simulink model "internal_system"  (R2022b)
settings: Solver=VariableStepAuto  StartTime=0.0  StopTime=600  RelTol=1e-3
model workspace (MAT data in the model file):
  F = 1
settings Model: Creator=aless  LastModifiedBy=aless
settings DebuggingCC: UnconnectedInputMsg=warning  UnconnectedOutputMsg=warning  UnconnectedLineMsg=warning
settings ModelReferenceCC: EnableRefExpFcnMdlSchedulingChecks=on
settings RTWCC: DLArmComputeVersion=19.05

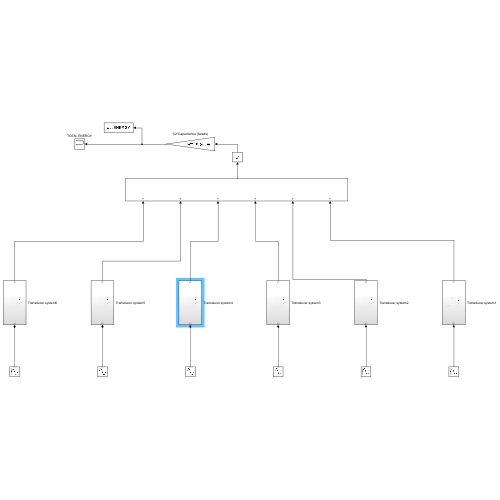
[thumbnail: Simulink's stored preview of the top-level diagram]
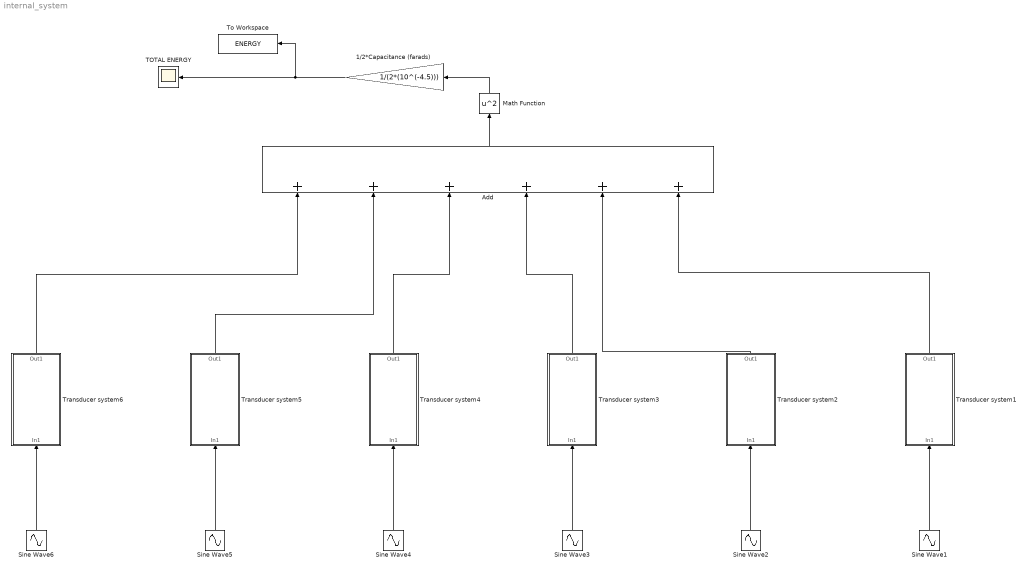
== system internal_system ==
  1/2*Capacitance (farads) : Gain  Gain=1/(2*(10^(-4.5)))
  Add : Sum  Inputs=++++++
  Math Function : Math  Operator=square
  Sine Wave1 : Sin  Amplitude=18670  Frequency=0.1176  SampleTime=0
  Sine Wave2 : Sin  Amplitude=18670  Frequency=0.1176  Phase=1/2  SampleTime=0
  Sine Wave3 : Sin  Amplitude=18670  Frequency=0.1176  Phase=1/3  SampleTime=0
  Sine Wave4 : Sin  Amplitude=18670  Frequency=0.1176  Phase=4/5  SampleTime=0
  Sine Wave5 : Sin  Amplitude=18670  Frequency=0.1176  Phase=1/5  SampleTime=0
  Sine Wave6 : Sin  Amplitude=18670  Frequency=0.1176  Phase=11/12  SampleTime=0
  TOTAL ENERGY : Scope
  To Workspace : ToWorkspace  VariableName=ENERGY  SaveFormat=Timeseries  SampleTime=-1
  Transducer system1 : Subsystem
  Transducer system2 : Subsystem
  Transducer system3 : Subsystem
  Transducer system4 : Subsystem
  Transducer system5 : Subsystem
  Transducer system6 : Subsystem
  wires:
  Sine Wave5/1 -> Transducer system5/1(In1)
  Sine Wave4/1 -> Transducer system4/1(In1)
  Sine Wave3/1 -> Transducer system3/1(In1)
  Sine Wave2/1 -> Transducer system2/1(In1)
  Sine Wave1/1 -> Transducer system1/1(In1)
  Transducer system6/1(Out1) -> Add/1
  Transducer system5/1(Out1) -> Add/2
  Transducer system4/1(Out1) -> Add/3
  Sine Wave6/1 -> Transducer system6/1(In1)
  Transducer system1/1(Out1) -> Add/6
  Transducer system2/1(Out1) -> Add/5
  Transducer system3/1(Out1) -> Add/4
  1/2*Capacitance (farads)/1 -> To Workspace/1, TOTAL ENERGY/1
  Add/1 -> Math Function/1
  Math Function/1 -> 1/2*Capacitance (farads)/1

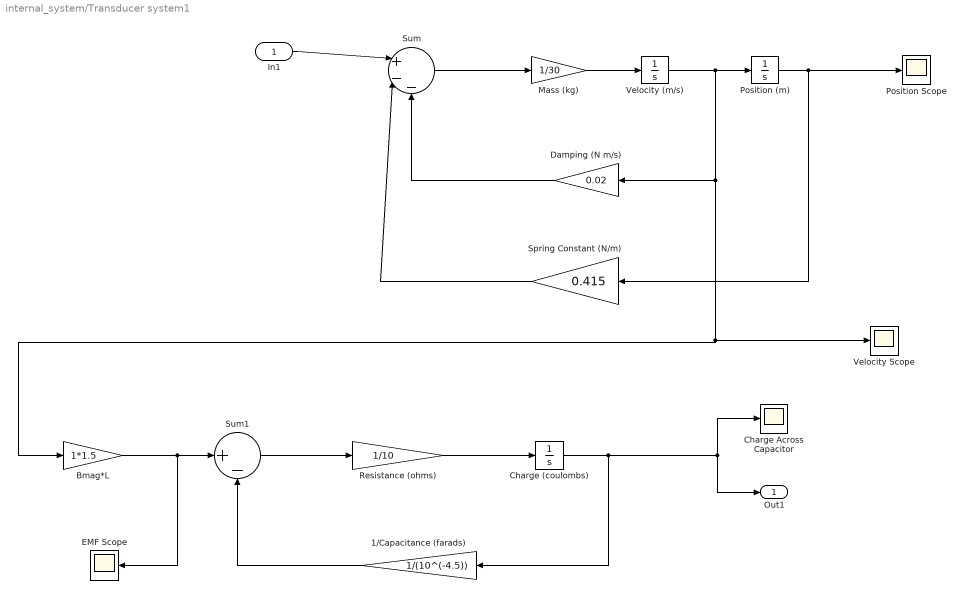
== system internal_system/Transducer system1 ==
  In1 : Inport
  1/Capacitance (farads) : Gain  Gain=1/(10^(-4.5))
  Bmag*L : Gain  Gain=1*1.5
  Charge (coulombs) : Integrator
  Charge Across Capacitor : Scope
  Damping (N m/s) : Gain  Gain=0.02
  EMF Scope : Scope
  Mass (kg) : Gain  Gain=1/30
  Position (m) : Integrator
  Position Scope : Scope
  Resistance (ohms) : Gain  Gain=1/10
  Spring Constant (N/m) : Gain  Gain=0.415
  Sum : Sum  Inputs=|+--
  Sum1 : Sum  Inputs=|+-
  Velocity (m/s) : Integrator
  Velocity Scope : Scope
  Out1 : Outport
  wires:
  Mass (kg)/1 -> Velocity (m/s)/1
  Sum/1 -> Mass (kg)/1
  Damping (N m/s)/1 -> Sum/3
  Position (m)/1 -> Position Scope/1, Spring Constant (N/m)/1
  Spring Constant (N/m)/1 -> Sum/2
  Velocity (m/s)/1 -> Damping (N m/s)/1, Bmag*L/1, Velocity Scope/1, Position (m)/1
  In1/1 -> Sum/1
  Sum1/1 -> Resistance (ohms)/1
  Bmag*L/1 -> EMF Scope/1, Sum1/1
  1/Capacitance (farads)/1 -> Sum1/2
  Resistance (ohms)/1 -> Charge (coulombs)/1
  Charge (coulombs)/1 -> 1/Capacitance (farads)/1, Out1/1, Charge Across Capacitor/1

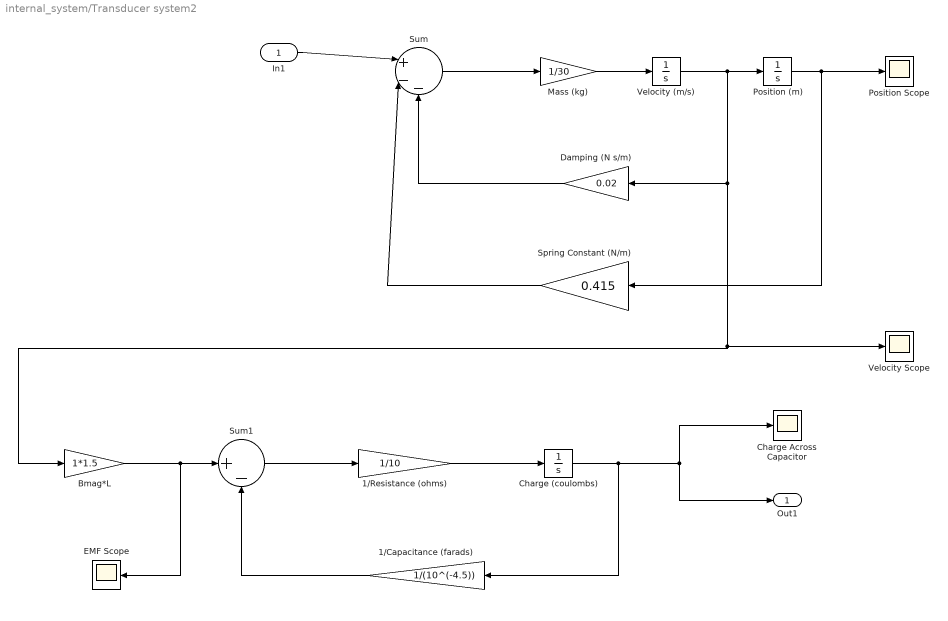
== system internal_system/Transducer system2 ==
  In1 : Inport
  1/Capacitance (farads) : Gain  Gain=1/(10^(-4.5))
  1/Resistance (ohms) : Gain  Gain=1/10
  Bmag*L : Gain  Gain=1*1.5
  Charge (coulombs) : Integrator
  Charge Across Capacitor : Scope
  Damping (N s/m) : Gain  Gain=0.02
  EMF Scope : Scope
  Mass (kg) : Gain  Gain=1/30
  Position (m) : Integrator
  Position Scope : Scope
  Spring Constant (N/m) : Gain  Gain=0.415
  Sum : Sum  Inputs=|+--
  Sum1 : Sum  Inputs=|+-
  Velocity (m/s) : Integrator
  Velocity Scope : Scope
  Out1 : Outport
  wires:
  Mass (kg)/1 -> Velocity (m/s)/1
  Sum/1 -> Mass (kg)/1
  Damping (N s/m)/1 -> Sum/3
  Position (m)/1 -> Position Scope/1, Spring Constant (N/m)/1
  Spring Constant (N/m)/1 -> Sum/2
  Velocity (m/s)/1 -> Damping (N s/m)/1, Bmag*L/1, Velocity Scope/1, Position (m)/1
  In1/1 -> Sum/1
  Sum1/1 -> 1/Resistance (ohms)/1
  Bmag*L/1 -> EMF Scope/1, Sum1/1
  1/Capacitance (farads)/1 -> Sum1/2
  1/Resistance (ohms)/1 -> Charge (coulombs)/1
  Charge (coulombs)/1 -> 1/Capacitance (farads)/1, Charge Across Capacitor/1, Out1/1

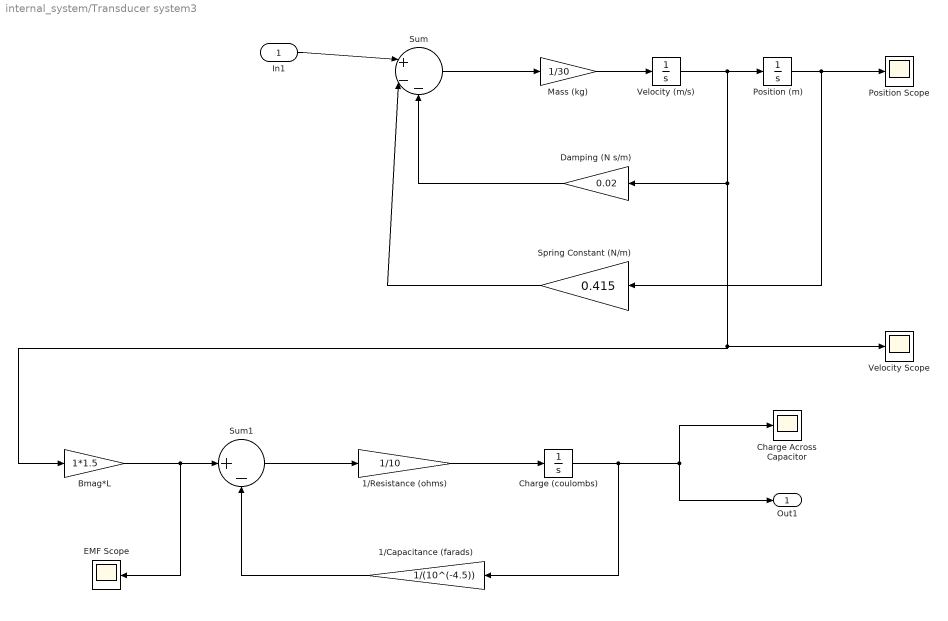
== system internal_system/Transducer system3 ==
  In1 : Inport
  1/Capacitance (farads) : Gain  Gain=1/(10^(-4.5))
  1/Resistance (ohms) : Gain  Gain=1/10
  Bmag*L : Gain  Gain=1*1.5
  Charge (coulombs) : Integrator
  Charge Across Capacitor : Scope
  Damping (N s/m) : Gain  Gain=0.02
  EMF Scope : Scope
  Mass (kg) : Gain  Gain=1/30
  Position (m) : Integrator
  Position Scope : Scope
  Spring Constant (N/m) : Gain  Gain=0.415
  Sum : Sum  Inputs=|+--
  Sum1 : Sum  Inputs=|+-
  Velocity (m/s) : Integrator
  Velocity Scope : Scope
  Out1 : Outport
  wires:
  Mass (kg)/1 -> Velocity (m/s)/1
  Sum/1 -> Mass (kg)/1
  Damping (N s/m)/1 -> Sum/3
  Position (m)/1 -> Position Scope/1, Spring Constant (N/m)/1
  Spring Constant (N/m)/1 -> Sum/2
  Velocity (m/s)/1 -> Damping (N s/m)/1, Bmag*L/1, Velocity Scope/1, Position (m)/1
  In1/1 -> Sum/1
  Sum1/1 -> 1/Resistance (ohms)/1
  Bmag*L/1 -> EMF Scope/1, Sum1/1
  1/Capacitance (farads)/1 -> Sum1/2
  1/Resistance (ohms)/1 -> Charge (coulombs)/1
  Charge (coulombs)/1 -> 1/Capacitance (farads)/1, Charge Across Capacitor/1, Out1/1

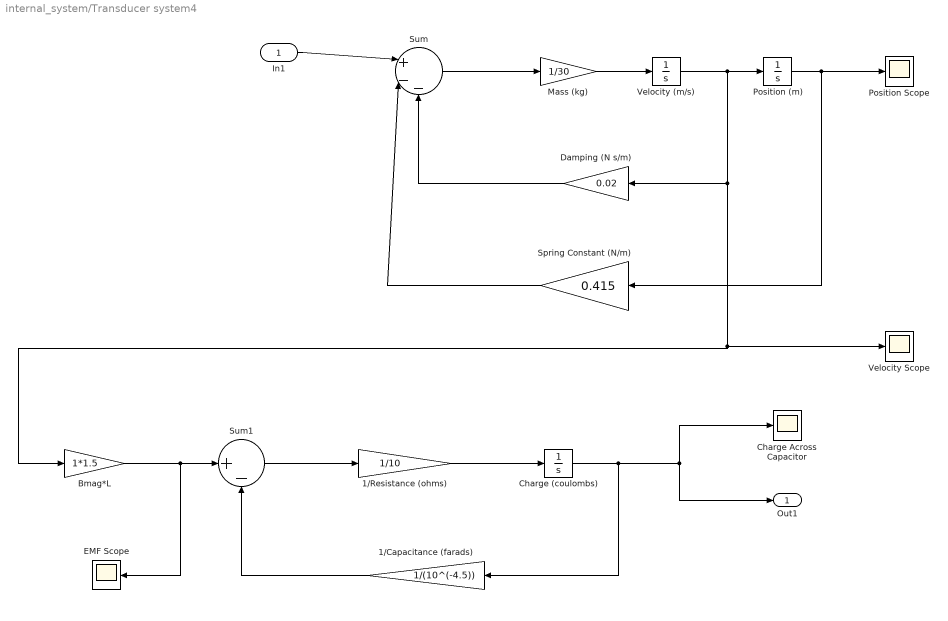
== system internal_system/Transducer system4 ==
  In1 : Inport
  1/Capacitance (farads) : Gain  Gain=1/(10^(-4.5))
  1/Resistance (ohms) : Gain  Gain=1/10
  Bmag*L : Gain  Gain=1*1.5
  Charge (coulombs) : Integrator
  Charge Across Capacitor : Scope
  Damping (N s/m) : Gain  Gain=0.02
  EMF Scope : Scope
  Mass (kg) : Gain  Gain=1/30
  Position (m) : Integrator
  Position Scope : Scope
  Spring Constant (N/m) : Gain  Gain=0.415
  Sum : Sum  Inputs=|+--
  Sum1 : Sum  Inputs=|+-
  Velocity (m/s) : Integrator
  Velocity Scope : Scope
  Out1 : Outport
  wires:
  Mass (kg)/1 -> Velocity (m/s)/1
  Sum/1 -> Mass (kg)/1
  Damping (N s/m)/1 -> Sum/3
  Position (m)/1 -> Position Scope/1, Spring Constant (N/m)/1
  Spring Constant (N/m)/1 -> Sum/2
  Velocity (m/s)/1 -> Damping (N s/m)/1, Bmag*L/1, Velocity Scope/1, Position (m)/1
  In1/1 -> Sum/1
  Sum1/1 -> 1/Resistance (ohms)/1
  Bmag*L/1 -> EMF Scope/1, Sum1/1
  1/Capacitance (farads)/1 -> Sum1/2
  1/Resistance (ohms)/1 -> Charge (coulombs)/1
  Charge (coulombs)/1 -> 1/Capacitance (farads)/1, Charge Across Capacitor/1, Out1/1

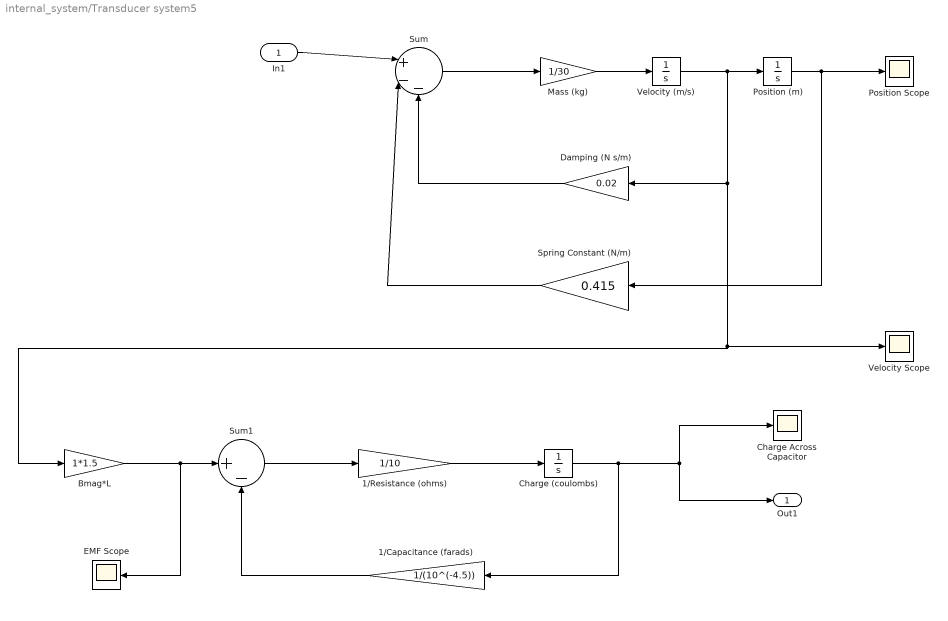
== system internal_system/Transducer system5 ==
  In1 : Inport
  1/Capacitance (farads) : Gain  Gain=1/(10^(-4.5))
  1/Resistance (ohms) : Gain  Gain=1/10
  Bmag*L : Gain  Gain=1*1.5
  Charge (coulombs) : Integrator
  Charge Across Capacitor : Scope
  Damping (N s/m) : Gain  Gain=0.02
  EMF Scope : Scope
  Mass (kg) : Gain  Gain=1/30
  Position (m) : Integrator
  Position Scope : Scope
  Spring Constant (N/m) : Gain  Gain=0.415
  Sum : Sum  Inputs=|+--
  Sum1 : Sum  Inputs=|+-
  Velocity (m/s) : Integrator
  Velocity Scope : Scope
  Out1 : Outport
  wires:
  Mass (kg)/1 -> Velocity (m/s)/1
  Sum/1 -> Mass (kg)/1
  Damping (N s/m)/1 -> Sum/3
  Position (m)/1 -> Position Scope/1, Spring Constant (N/m)/1
  Spring Constant (N/m)/1 -> Sum/2
  Velocity (m/s)/1 -> Damping (N s/m)/1, Bmag*L/1, Velocity Scope/1, Position (m)/1
  In1/1 -> Sum/1
  Sum1/1 -> 1/Resistance (ohms)/1
  Bmag*L/1 -> EMF Scope/1, Sum1/1
  1/Capacitance (farads)/1 -> Sum1/2
  1/Resistance (ohms)/1 -> Charge (coulombs)/1
  Charge (coulombs)/1 -> 1/Capacitance (farads)/1, Charge Across Capacitor/1, Out1/1

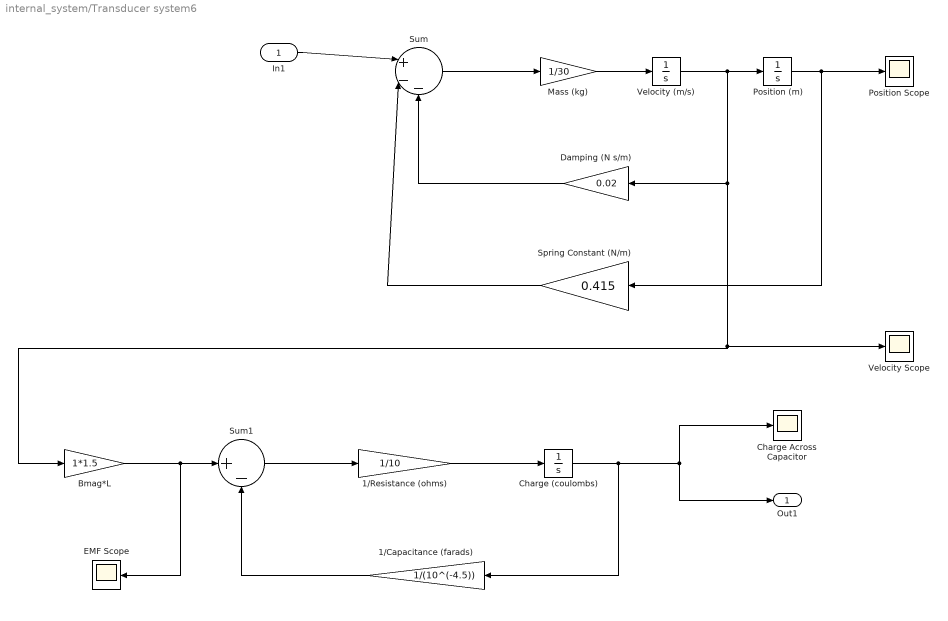
== system internal_system/Transducer system6 ==
  In1 : Inport
  1/Capacitance (farads) : Gain  Gain=1/(10^(-4.5))
  1/Resistance (ohms) : Gain  Gain=1/10
  Bmag*L : Gain  Gain=1*1.5
  Charge (coulombs) : Integrator
  Charge Across Capacitor : Scope
  Damping (N s/m) : Gain  Gain=0.02
  EMF Scope : Scope
  Mass (kg) : Gain  Gain=1/30
  Position (m) : Integrator
  Position Scope : Scope
  Spring Constant (N/m) : Gain  Gain=0.415
  Sum : Sum  Inputs=|+--
  Sum1 : Sum  Inputs=|+-
  Velocity (m/s) : Integrator
  Velocity Scope : Scope
  Out1 : Outport
  wires:
  Mass (kg)/1 -> Velocity (m/s)/1
  Sum/1 -> Mass (kg)/1
  Damping (N s/m)/1 -> Sum/3
  Position (m)/1 -> Position Scope/1, Spring Constant (N/m)/1
  Spring Constant (N/m)/1 -> Sum/2
  Velocity (m/s)/1 -> Damping (N s/m)/1, Bmag*L/1, Velocity Scope/1, Position (m)/1
  In1/1 -> Sum/1
  Sum1/1 -> 1/Resistance (ohms)/1
  Bmag*L/1 -> EMF Scope/1, Sum1/1
  1/Capacitance (farads)/1 -> Sum1/2
  1/Resistance (ohms)/1 -> Charge (coulombs)/1
  Charge (coulombs)/1 -> 1/Capacitance (farads)/1, Charge Across Capacitor/1, Out1/1
